simulink library "Pressure_Drop_Collector"  (R2018b)
settings: Solver=ode45  StartTime=0.0  StopTime=10.0  RelTol=1e-3  EnableMultiTasking=on
libraries: carnot x2, simulink_extras x1
settings Model: Creator=drhf  LastModifiedBy=P41573
settings DataIOCC: LimitDataPoints=on  SaveFormat=Array  SignalLoggingSaveFormat=ModelDataLogs
settings OptimizationCC: ExpressionDepthLimit=2147483647  LifeSpan=inf
settings DebuggingCC: UnderspecifiedInitializationDetection=Classic  MergeDetectMultiDrivingBlocksExec=none  SolverPrmCheckMsg=warning  FcnCallInpInsideContextMsg=warning  StateNameClashWarn=warning  SFUnexpectedBacktrackingDiag=warning  SFNoUnconditionalDefaultTransitionDiag=warning  SFExecutionAtInitializationDiag=none
settings HardwareCC: ProdBitPerPointer=32  ProdBitPerSizeT=32  ProdBitPerPtrDiffT=32  ProdLargestAtomicFloat=None  ProdIntDivRoundTo=Undefined  ProdEndianess=Unspecified  ProdWordSize=32  ProdHWDeviceType=32-bit Generic
settings ModelReferenceCC: PropagateSignalLabelsOutOfModel=off
settings SFSimCC: SimUseLocalCustomCode=off
settings RTWCC: RTWUseLocalCustomCode=off
settings CodeAppCC: StateflowObjectComments=on
settings GRTTargetCC: TargetLangStandard=C89/C90 (ANSI)  GeneratePreprocessorConditionals=Disable all  CombineOutputUpdateFcns=off  GRTInterface=on
settings ConfigComp: CovMetricSettings=dw  CovHtmlReporting=on  CovSaveCumulativeToWorkspaceVar=on  CovSaveSingleToWorkspaceVar=on  CovExternalEMLEnable=off

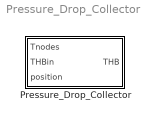
== system Pressure_Drop_Collector ==
  Pressure_Drop_Collector : Subsystem  mask(Pressure Drop Collector){len=1, lin=100, qua=100}
      mask prompts: len "Length of collector in m"; lin "l : linear pressure drop Pa/(kg/s)"; qua "q : quadratic pressure drop Pa/(kg/s)²"
      mask help:
      | Calculates the pressure drop according to constant values of con, lin and qua:
      | dp_dyn = c + l*mdot + q*mdot²
      | Static height is taken in account via the collector inclination, the length and the temperatures:
      | dp_stat = density * grav * height
      | Total pressure is dp = dp_dyn + dpstat
      mask Help: web(fullfile(path_carnot('help'),'Pressure_Drop_Collector.html'),'-helpbrowser')
      mask TypeOptions len: Gain/Gain
      mask TypeOptions lin: Pressure_Drop_Fix/lin
      mask TypeOptions qua: Pressure_Drop_Fix/qua

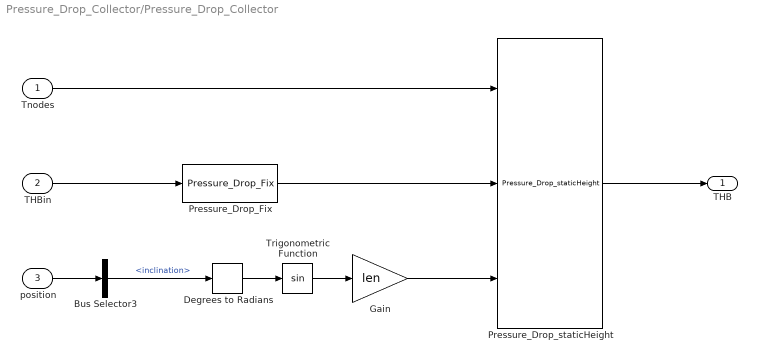
== system Pressure_Drop_Collector/Pressure_Drop_Collector ==
  Tnodes : Inport
  THBin : Inport  Port=2
  position : Inport  Port=3
  Bus Selector3 : BusSelector  OutputSignals=inclination
  Degrees to Radians : simulink_extras/Transformations/Degrees to Radians
  Gain : Gain  Gain=len
  Pressure_Drop_Fix : carnot/Basic/Pressure_Drop/Pressure_Drop_Fix  con=0  lin=lin  qua=qua
      settings: SourceProductName=Carnot
  Pressure_Drop_staticHeight : carnot/Basic/Pressure_Drop/Pressure_Drop_staticHeight
      settings: SourceProductName=Carnot
  Trigonometric Function : Trigonometry
  THB : Outport
  wires:
  Gain/1 -> Pressure_Drop_staticHeight/3
  Bus Selector3/1 -> Degrees to Radians/1  "<inclination>"
  position/1 -> Bus Selector3/1
  Trigonometric Function/1 -> Gain/1
  THBin/1 -> Pressure_Drop_Fix/1
  Pressure_Drop_Fix/1 -> Pressure_Drop_staticHeight/2
  Tnodes/1 -> Pressure_Drop_staticHeight/1
  Pressure_Drop_staticHeight/1 -> THB/1
  Degrees to Radians/1 -> Trigonometric Function/1
